simulink model "LED_Cmd_varZ"  (Simulink 7.9)
settings: Solver=FixedStepDiscrete  StartTime=0.0  StopTime=10  RelTol=1e-3  SampleTimeConstraint=STIndependent
PreLoadFcn:
  | LED_Cmd_varZ_selfinit
libraries: simulink x2
CloseFcn:
  | rtwprivate ssgencode ModelCloseRequest ADL
settings Model: RequirementInfo="{}  %GIDa_ffb28f1c_3982_4734_9f04_bbd4c8d0ce22"  MinMaxOverflowLogging=ForceOff  Creator=fguerin  LastModifiedBy=klindqvi  CovMetricSettings=dcme  CovHtmlReporting=off  covSaveCumulativeToWorkspaceVar=off  CovSaveSingleToWorkspaceVar=off  CovModelRefEnable=off  CovExternalEMLEnable=on
settings DataIOCC: ExternalInput=SIM_LockDoorRequest  LimitDataPoints=off  SaveOutput=off  DSMLogging=off  SaveTime=off  SignalLoggingName=logsOut
settings OptimizationCC: InlineParams=on  InlineInvariantSignals=on  EnhancedBackFolding=on  ZeroExternalMemoryAtStartup=off  ZeroInternalMemoryAtStartup=off  EfficientFloat2IntCast=on  OptimizeModelRefInitCode=on  LifeSpan=1
settings DebuggingCC: ReadBeforeWriteMsg=EnableAllAsError  WriteAfterWriteMsg=EnableAllAsError  WriteAfterReadMsg=EnableAllAsError  AlgebraicLoopMsg=error  ArtificialAlgebraicLoopMsg=error  SaveWithDisabledLinksMsg=error  SaveWithParameterizedLinksMsg=error  CheckSSInitialOutputMsg=off  CheckExecutionContextPreStartOutputMsg=on  CheckExecutionContextRuntimeOutputMsg=on  BlockPriorityViolationMsg=error  SolverPrmCheckMsg=none  MultiTaskCondExecSysMsg=warning  MultiTaskRateTransMsg=warning  IntegerOverflowMsg=none  ParameterUnderflowMsg=error  ParameterPrecisionLossMsg=error  ParameterTunabilityLossMsg=error  UnnecessaryDatatypeConvMsg=warning  VectorMatrixConversionMsg=error  SignalLabelMismatchMsg=warning  SFcnCompatibilityMsg=error  BusObjectLabelMismatch=error  RootOutportRequireBusObject=error  AssertControl=DisableAll  ModelReferenceIOMsg=error  ModelReferenceIOMismatchMessage=error  ModelReferenceCSMismatchMessage=warning  UnknownTsInhSupMsg=error  ModelReferenceDataLoggingMessage=error  ModelReferenceSymbolNameMessage=none  StrictBusMsg=ErrorOnBusTreatedAsVector
settings HardwareCC: ProdLargestAtomicInteger=Long  ProdLargestAtomicFloat=Double  ProdIntDivRoundTo=Zero  ProdEndianess=BigEndian  ProdHWDeviceType=Freescale->MPC5500
settings ModelReferenceCC: ModelReferenceNumInstancesAllowed=Single
settings SFSimCC: SimParseCustomCode=off
settings RTWCC: SystemTargetFile=ert.tlc  TemplateMakefile=ert_default_tmf  Description=Embedded Coder  GenerateReport=on  RTWVerbose=off  ProcessScript=ert_make_rtw_hook  IncludeHyperlinkInReport=on  GenerateTraceInfo=on  GenerateTraceReport=on  GenerateTraceReportSl=on  GenerateTraceReportSf=on  GenerateTraceReportEml=on  GenerateCodeMetricsReport=on
settings MATStruct: className=rtw.pil.Bullseye  argsAllComponents=[]  excludedModels=[]  includeReferencedModels=on  includeTopModel=on  enabled=off
settings CodeAppCC: ForceParamTrailComments=on  IgnoreCustomStorageClasses=off  IgnoreTestpoints=on  MangleLength=4  InlinedPrmAccess=Macros  ReqsInCode=on
settings ERTTargetCC: CodeReplacementLibrary=ANSI_C  MultiwordLength=2048  SupportAbsoluteTime=off  SupportNonFinite=off  SupportComplex=off  PortableWordSizes=on  InlinedParameterPlacement=NonHierarchical  ERTCustomFileTemplate=example_file_process.tlc  ConvertIfToSwitch=off  SuppressUnreachableDefaultCases=off
settings ConfigComp: Description=Design Verifier Custom Configuration Component  DVMaxProcessTime=600  DVDisplayUnsatisfiableObjectives=on  DVAutomaticStubbing=off  DVOutputDir=C:\work\Presentations\ISO26262_workshop\newsandbox\iso26262package\WorkProducts\CodeTest  DVMakeOutputFilesUnique=off  DVModelCoverageObjectives=MCDC  DVTestSuiteOptimization=CombinedObjectives  DVDataFileName=LED_Cmd_varZ_sldvdata.mat  DVHarnessModelFileName=C:\work\Presentations\ISO26262_workshop\newsandbox\iso26262package\WorkProducts\CodeTest\LED_Cmd_varZ_eqHarness  DVModelReferenceHarness=on  DVSaveReport=on  DVReportFileName=LED_Cmd_varZ_SLDV.html  DVDisplayReport=off

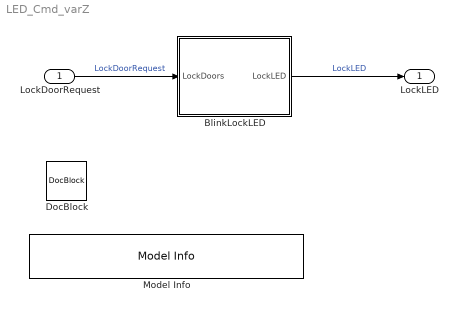
== system LED_Cmd_varZ ==
  LockDoorRequest : Inport  OutDataTypeStr=boolean  PortDimensions=1
  BlinkLockLED : Stateflow chart  RequirementInfo={'other' '..\doorlockingsystem_swr.doc' '@Simulink_requirement_item_4' 'true' 'REQ202 – The lock mechanism should indicate the state. A locked state should be indicated by a flashing light and an unlocked state by no light.' '' } %GIDa_2fa83fc7_e887_441b_a127_89ab2a7e14b5  TreatAsAtomicUnit=on
  DocBlock : simulink/Model-Wide Utilities/DocBlock  DocumentType=Text
  Model Info : simulink/Model-Wide Utilities/Model Info  InitialSaveTempField=klindqvi#|#2012-01-18 22:25:05 +0100 (on, 18 jan 2012)#|#69#|#file://mathworks/se/SalesService/Pilot_Engineering/Projects/PSP-ISO26262Workshop/repository/system/C_DoorLock/F_Actuator_Ctrl/LED_Cmd_varZ.mdl 69 2012-01-18 21:25:05Z klindqvi#|#LED_Cmd_varZ.mdl 69 2012-01-18 21:25:05Z klindqvi#|##|##|##|##|#  InitialBlockCM=RCS  BlockCM=RCS  Frame=on  SaveTempField=klindqvi#|#2012-01-18 22:25:05 +0100 (on, 18 jan 2012)#|#69#|#file://mathworks/se/SalesService/Pilot_Engineering/Projects/PSP-ISO26262Workshop/repository/system/C_DoorLock/F_Actuator_Ctrl/LED_Cmd_varZ.mdl 69 2012-01-18 21:25:05Z klindqvi#|#LED_Cmd_varZ.mdl 69 2012-01-18 21:25:05Z klindqvi#|##|##|##|##|#  DisplayStringWithTags=|  HorizontalTextAlignment=Center  LeftAlignmentValue=0.5  SourceBlockDiagram=LED_Cmd_varZ  TagMaxNumber=20  CMTag1=$Author: klindqvi $  CMTag2=$Date: 2012-03-09 09:14:38 +0000 (Fri, 09 Mar 2012) $  CMTag3=$Revision: 84 $  CMTag4=$Header: file://mathworks/se/SalesService/Pilot_Engineering/Projects/PSP-ISO26262Workshop/repository/trunk/system/C_DoorLock/F_Actuator_Ctrl/LED_Cmd_varZ.mdl 84 2012-03-09 09:14:38Z klindqvi $  CMTag5=$Id: LED_Cmd_varZ.mdl 84 2012-03-09 09:14:38Z klindqvi $  CMTag6=$Locker: $  CMTag7=$RCSfile: $  CMTag8=$Source: $  CMTag9=$State: $
      | %<Author>
      | %<Revision>
      | %<Date>
  LockLED : Outport  OutDataTypeStr=boolean  PortDimensions=1
  wires:
  LockDoorRequest/1 -> BlinkLockLED/1(LockDoors)  "LockDoorRequest"
  BlinkLockLED/1(LockLED) -> LockLED/1  "LockLED"

== stateflow chart BlinkLockLED ==
  state Doors_Unlock
    entry: LockLED = 0;
  state Doors_Lock
    entry: LockLED = 1;
    during: LockLED = Blink(LockLED);
  state y = Blink(x) [function]
    (default) -> (junction 6)
    (junction 6) -> (junction 7) [order 1] : [ x == 1]
    (junction 6) -> (junction 8) [order 2] : {y = 1;}
    (junction 7) -> (junction 8) : {y = 0;}
  Doors_Unlock -> Doors_Lock : [LockDoors]
  Doors_Lock -> Doors_Unlock : [!LockDoors]
  (default) -> Doors_Unlock
  data: x function_input double; y function_output double; LockDoors input double; LockLED output double
